simulink model "mass_spring_damper_sim"  (R2018a)
settings: Solver=ode45  StartTime=0.0  StopTime=10000  MaxStep=0.1  RelTol=1e-3
undefined symbols (not defined in the file or in its folder): mass_spring_damper_animation
libraries: simulink x1
settings Model: Creator=canla  LastModifiedBy=canla
settings OptimizationCC: LifeSpan=inf

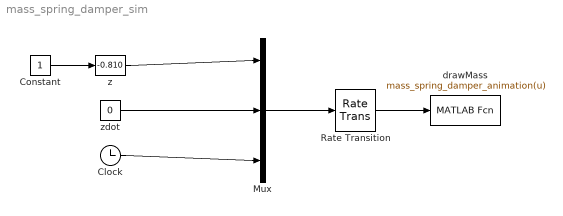
== system mass_spring_damper_sim ==
  Clock : Clock
  Constant : Constant
  Mux : Mux  Inputs=3
  Rate Transition : RateTransition
  drawMass : MATLABFcn  MATLABFcn=mass_spring_damper_animation(u)  OutputDimensions=0
  "z " : simulink/Math Operations/Slider Gain  gain=-0.810  low=-1.5  high=1.5
  zdot : Constant  Value=0
  wires:
  Mux/1 -> Rate Transition/1
  Clock/1 -> Mux/3
  Rate Transition/1 -> drawMass/1
  "z "/1 -> Mux/1
  Constant/1 -> "z "/1
  zdot/1 -> Mux/2
